simulink model "Differential_MP_CS9"  (Simulink 7.6)
settings: Solver=ode45  SolverMode=SingleTasking  StartTime=0  StopTime=20  FixedStep=0.002  RelTol=1e-3  AbsTol=1e-6
libraries: Solver_SF x1
settings Model: Creator=jhu  LastModifiedBy=hkawanishi  ExtModeTrigMode=oneshot  ExtModeArmWhenConnect=off
settings DataIOCC: LimitDataPoints=off  SignalLoggingName=sigsOut
settings OptimizationCC: BooleanDataType=off
settings DebuggingCC: SaveWithParameterizedLinksMsg=none  SignalResolutionControl=TryResolveAllWithWarning  SolverPrmCheckMsg=none  MultiTaskDSMMsg=warning  MultiTaskCondExecSysMsg=none  FcnCallInpInsideContextMsg=Enable All  StateNameClashWarn=none
settings HardwareCC: TargetUnknown=on
settings RTWCC: TemplateMakefile=grt_vc.tmf  IncludeERTFirstTime=on
settings CodeAppCC: CustomSymbolStrType=$N$R$M_T

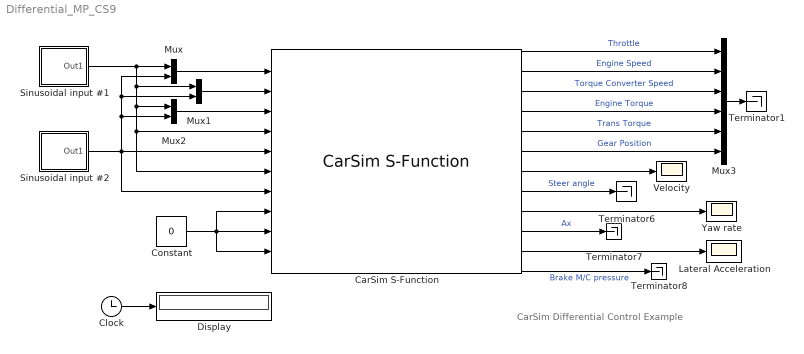
== system Differential_MP_CS9 ==
  note: CarSim Differential Control Example
  CarSim S-Function : Solver_SF/CarSim S-Function  Priority=1  SIMFILE=simfile.sim
  Clock : Clock
      settings: Decimation=10
  Constant : Constant  Value=0
  Display : Display
      settings: Format=bank  Decimation=100
  Lateral Acceleration : Scope
      settings: TickLabels=on  YMin=-1  YMax=1  DataFormat=Array  SampleTime=100
  Mux : Mux  Inputs=2
  Mux1 : Mux  Inputs=2
  Mux2 : Mux  Inputs=2
  Mux3 : Mux  Inputs=6
  Sinusoidal input #1 : Subsystem
  Sinusoidal input #2 : Subsystem
  Terminator{1,6..8} (4 alike) : Terminator
  Velocity : Scope
      settings: TickLabels=on  YMin=0  YMax=200  DataFormat=Array  SampleTime=100
  Yaw rate : Scope
      settings: TickLabels=on  YMin=-20  YMax=20  DataFormat=Array  SampleTime=100
  wires:
  Sinusoidal input #1/1(Out1) -> Mux/1, Mux2/1, CarSim S-Function/6, CarSim S-Function/4, Mux1/1
  CarSim S-Function/9 -> Yaw rate/1
  CarSim S-Function/11 -> Lateral Acceleration/1
  CarSim S-Function/1 -> Mux3/1  "Throttle"
  CarSim S-Function/4 -> Mux3/4  "Engine Torque"
  CarSim S-Function/5 -> Mux3/5  "Trans Torque"
  CarSim S-Function/6 -> Mux3/6  "Gear Position"
  CarSim S-Function/3 -> Mux3/3  "Torque Converter Speed"
  CarSim S-Function/2 -> Mux3/2  "Engine Speed"
  CarSim S-Function/8 -> Terminator6/1  "Steer angle"
  CarSim S-Function/10 -> Terminator7/1  "Ax"
  CarSim S-Function/12 -> Terminator8/1  "Brake M/C pressure"
  Clock/1 -> Display/1
  Mux/1 -> CarSim S-Function/1
  Sinusoidal input #2/1(Out1) -> Mux2/2, Mux/2, Mux1/2, CarSim S-Function/7, CarSim S-Function/5
  Mux2/1 -> CarSim S-Function/3
  CarSim S-Function/7 -> Velocity/1
  Mux3/1 -> Terminator1/1
  Constant/1 -> CarSim S-Function/9, CarSim S-Function/8, CarSim S-Function/10
  Mux1/1 -> CarSim S-Function/2

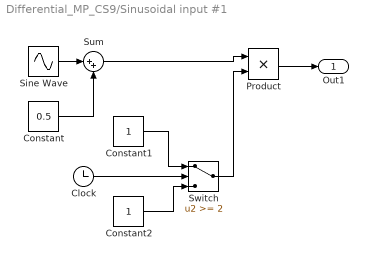
== system Differential_MP_CS9/Sinusoidal input #1 ==
  Clock : Clock
      settings: Decimation=10
  Constant : Constant  Value=0.5
  Constant1 : Constant
  Constant2 : Constant
  Product : Product  SaturateOnIntegerOverflow=on  InputSameDT=on  OutDataTypeStr=Inherit: Same as first input
  Sine Wave : Sin  Amplitude=0.5  Frequency=0.25*2*pi  Phase=3/2*pi  SampleTime=0
  Sum : Sum  Inputs=|++  SaturateOnIntegerOverflow=on  InputSameDT=on  OutDataTypeStr=Inherit: Same as first input
  Switch : Switch  Threshold=2  SaturateOnIntegerOverflow=on  InputSameDT=on
  Out1 : Outport
  wires:
  Sine Wave/1 -> Sum/1
  Constant/1 -> Sum/2
  Clock/1 -> Switch/2
  Constant1/1 -> Switch/1
  Constant2/1 -> Switch/3
  Switch/1 -> Product/2
  Product/1 -> Out1/1
  Sum/1 -> Product/1

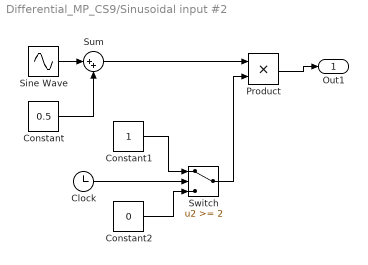
== system Differential_MP_CS9/Sinusoidal input #2 ==
  Clock : Clock
      settings: Decimation=10
  Constant : Constant  Value=0.5
  Constant1 : Constant
  Constant2 : Constant  Value=0
  Product : Product  SaturateOnIntegerOverflow=on  InputSameDT=on  OutDataTypeStr=Inherit: Same as first input
  Sine Wave : Sin  Amplitude=0.5  Frequency=0.25*2*pi  Phase=1/2*pi  SampleTime=0
  Sum : Sum  Inputs=|++  SaturateOnIntegerOverflow=on  InputSameDT=on  OutDataTypeStr=Inherit: Same as first input
  Switch : Switch  Threshold=2  SaturateOnIntegerOverflow=on  InputSameDT=on
  Out1 : Outport
  wires:
  Sine Wave/1 -> Sum/1
  Constant/1 -> Sum/2
  Clock/1 -> Switch/2
  Sum/1 -> Product/1
  Constant1/1 -> Switch/1
  Constant2/1 -> Switch/3
  Switch/1 -> Product/2
  Product/1 -> Out1/1
